simulink model "AE_315__W4__Mass_Spring_damper_TF"  (R2023a)
settings: Solver=VariableStepAuto  StartTime=0.0  StopTime=10.0  RelTol=1e-3
settings Model: Creator=zeyadmanaa  LastModifiedBy=zeyadmanaa

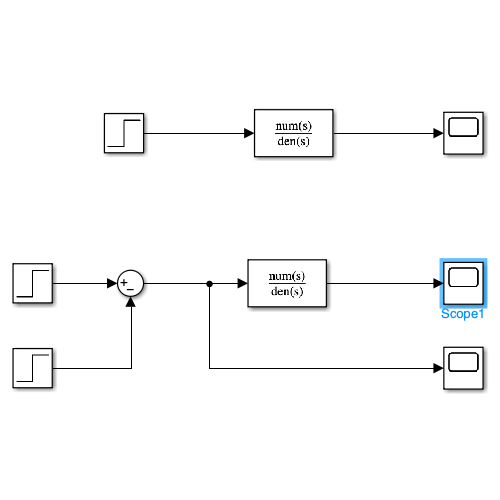
[thumbnail: Simulink's stored preview of the top-level diagram]
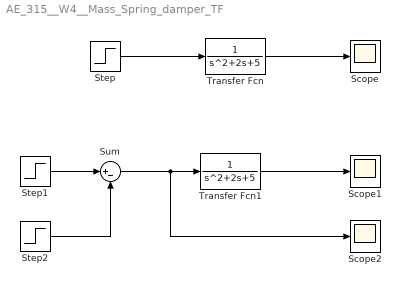
== system AE_315__W4__Mass_Spring_damper_TF ==
  Scope : Scope
  Scope1 : Scope
  Scope2 : Scope
  Step : Step  SampleTime=0
  Step1 : Step  Time=0  SampleTime=0
  Step2 : Step  Time=0.01  Before=00  SampleTime=0
  Sum : Sum  Inputs=|+-
  Transfer Fcn : TransferFcn  Denominator=[1 2 5]
  Transfer Fcn1 : TransferFcn  Denominator=[1 2 5]
  wires:
  Step/1 -> Transfer Fcn/1
  Transfer Fcn/1 -> Scope/1
  Transfer Fcn1/1 -> Scope1/1
  Sum/1 -> Scope2/1, Transfer Fcn1/1
  Step1/1 -> Sum/1
  Step2/1 -> Sum/2
